simulink model "subsistema_trolley"  (R2023b)
settings: Solver=VariableStepAuto  StartTime=0.0  StopTime=10.0  RelTol=1e-3
undefined symbols (not defined in the file): bt, btb, btd, btm, btw, it, Jtd, Jtm_tb, Ktw, Mt, rtd, titatm_0, Ttb_Max, vt_0, wtm_0, xt_0, xtd_0
settings Model: Creator=nahue  LastModifiedBy=nahue

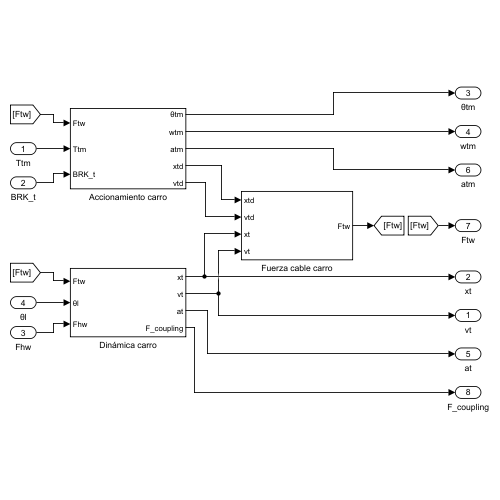
[thumbnail: Simulink's stored preview of the top-level diagram]
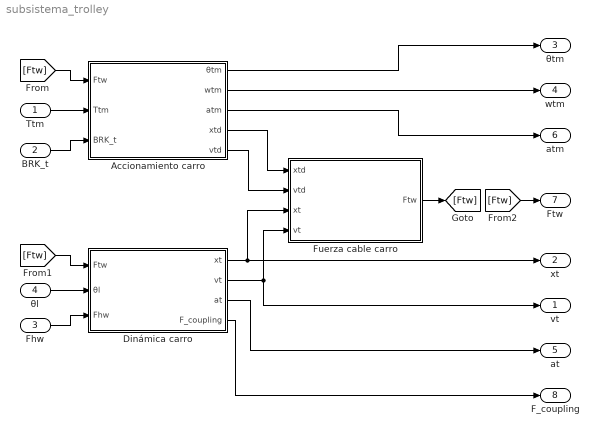
== system subsistema_trolley ==
  Ttm : Inport
  BRK_t : Inport  Port=2
  Fhw : Inport  Port=3
  θl : Inport  Port=4
  Accionamiento carro : Subsystem
  Dinámica carro : Subsystem
  Fuerza cable carro : Subsystem
  vt : Outport
  xt : Outport  Port=2
  θtm : Outport  Port=3
  wtm : Outport  Port=4
  at : Outport  Port=5
  atm : Outport  Port=6
  Ftw : Outport  Port=7
  F_coupling : Outport  Port=8
  wires:
  Ttm/1 -> Accionamiento carro/2(Ttm)
  BRK_t/1 -> Accionamiento carro/3(BRK_t)
  θl/1 -> Dinámica carro/2(θl)
  Fhw/1 -> Dinámica carro/3(Fhw)
  [Ftw] -> Accionamiento carro/1(Ftw)
  [Ftw] -> Dinámica carro/1(Ftw)
  Accionamiento carro/5(vtd) -> Fuerza cable carro/2(vtd)
  Dinámica carro/1(xt) -> xt/1, Fuerza cable carro/3(xt)
  Dinámica carro/2(vt) -> vt/1, Fuerza cable carro/4(vt)
  Fuerza cable carro/1(Ftw) -> [Ftw]
  Accionamiento carro/4(xtd) -> Fuerza cable carro/1(xtd)
  Accionamiento carro/2(wtm) -> wtm/1
  Accionamiento carro/1(θtm) -> θtm/1
  Dinámica carro/3(at) -> at/1
  Accionamiento carro/3(atm) -> atm/1
  [Ftw] -> Ftw/1
  Dinámica carro/4(F_coupling) -> F_coupling/1

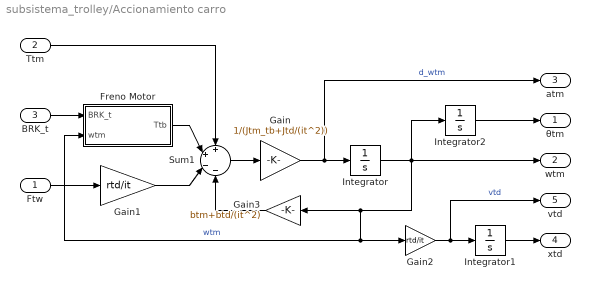
== system subsistema_trolley/Accionamiento carro ==
  Ftw : Inport
  Ttm : Inport  Port=2
  BRK_t : Inport  Port=3
  Freno Motor : Subsystem
  Gain : Gain  Gain=1/(Jtm_tb+Jtd/(it^2))
  Gain1 : Gain  Gain=rtd/it
  Gain2 : Gain  Gain=rtd/it
  Gain3 : Gain  Gain=btm+btd/(it^2)
  Integrator : Integrator  InitialCondition=wtm_0
  Integrator1 : Integrator  InitialCondition=xtd_0
  Integrator2 : Integrator  InitialCondition=titatm_0
  Sum1 : Sum  Inputs=++--
  θtm : Outport
  wtm : Outport  Port=2
  atm : Outport  Port=3
  xtd : Outport  Port=4
  vtd : Outport  Port=5
  wires:
  Sum1/1 -> Gain/1
  Integrator/1 -> Gain2/1, Freno Motor/2(wtm), Gain3/1, Integrator2/1, wtm/1  "wtm"
  Gain2/1 -> Integrator1/1, vtd/1  "vtd"
  Ttm/1 -> Sum1/1
  Gain/1 -> atm/1, Integrator/1  "d_wtm"
  BRK_t/1 -> Freno Motor/1(BRK_t)
  Integrator1/1 -> xtd/1
  Ftw/1 -> Gain1/1
  Gain1/1 -> Sum1/3
  Freno Motor/1(Ttb) -> Sum1/2
  Gain3/1 -> Sum1/4
  Integrator2/1 -> θtm/1

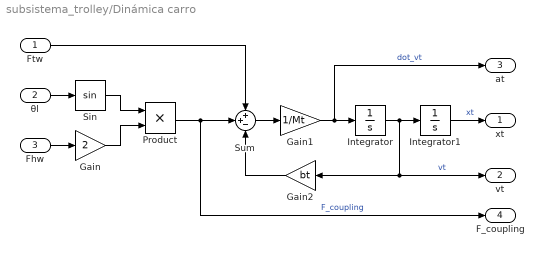
== system subsistema_trolley/Dinámica carro ==
  Ftw : Inport
  θl : Inport  Port=2
  Fhw : Inport  Port=3
  Gain : Gain  Gain=2
  Gain1 : Gain  Gain=1/Mt
  Gain2 : Gain  Gain=bt
  Integrator : Integrator  InitialCondition=vt_0
  Integrator1 : Integrator  InitialCondition=xt_0
  Product : Product
  Sin : Trigonometry
  Sum : Sum  Inputs=++-
  xt : Outport
  vt : Outport  Port=2
  at : Outport  Port=3
  F_coupling : Outport  Port=4
  wires:
  Gain1/1 -> at/1, Integrator/1  "dot_vt"
  Integrator/1 -> Gain2/1, vt/1, Integrator1/1  "vt"
  Gain2/1 -> Sum/3
  Sum/1 -> Gain1/1
  Integrator1/1 -> xt/1  "xt"
  Fhw/1 -> Gain/1
  Gain/1 -> Product/2
  θl/1 -> Sin/1
  Sin/1 -> Product/1
  Product/1 -> F_coupling/1, Sum/2  "F_coupling"
  Ftw/1 -> Sum/1

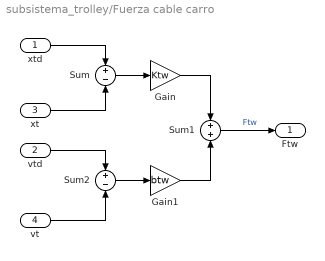
== system subsistema_trolley/Fuerza cable carro ==
  xtd : Inport
  vtd : Inport  Port=2
  xt : Inport  Port=3
  vt : Inport  Port=4
  Gain : Gain  Gain=Ktw
  Gain1 : Gain  Gain=btw
  Sum : Sum  Inputs=+-
  Sum1 : Sum
  Sum2 : Sum  Inputs=+-
  Ftw : Outport
  wires:
  xtd/1 -> Sum/1
  Gain1/1 -> Sum1/2
  Sum/1 -> Gain/1
  xt/1 -> Sum/2
  Sum2/1 -> Gain1/1
  Gain/1 -> Sum1/1
  vt/1 -> Sum2/2
  Sum1/1 -> Ftw/1  "Ftw"
  vtd/1 -> Sum2/1

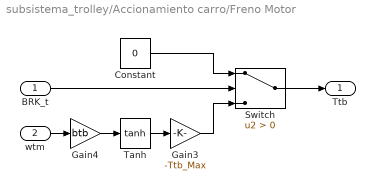
== system subsistema_trolley/Accionamiento carro/Freno Motor ==
  BRK_t : Inport
  wtm : Inport  Port=2
  Constant : Constant  Value=0
  Gain3 : Gain  Gain=-Ttb_Max
  Gain4 : Gain  Gain=btb
  Switch : Switch  Criteria=u2 > Threshold  SaturateOnIntegerOverflow=off  InputSameDT=off
  Tanh : Trigonometry  Operator=tanh
  Ttb : Outport
  wires:
  BRK_t/1 -> Switch/2
  Constant/1 -> Switch/1
  wtm/1 -> Gain4/1
  Gain4/1 -> Tanh/1
  Tanh/1 -> Gain3/1
  Gain3/1 -> Switch/3
  Switch/1 -> Ttb/1
